simulink model "LMS0"  (R2018a)
settings: Solver=FixedStepDiscrete  StartTime=0.0  StopTime=3  RelTol=1e-3  EnableMultiTasking=on
libraries: dspvision x4
settings Model: Creator=gianc  LastModifiedBy=gianc
settings DataIOCC: LimitDataPoints=on  SaveOutput=off  SignalLogging=off  SaveTime=off
settings OptimizationCC: LifeSpan=inf
settings DebuggingCC: AlgebraicLoopMsg=error  SingleTaskRateTransMsg=error  AllowSymbolicDim=off  SFUnexpectedBacktrackingDiag=warning  SFNoUnconditionalDefaultTransitionDiag=warning  SFExecutionAtInitializationDiag=none
settings CodeAppCC: StateflowObjectComments=on
settings GRTTargetCC: TargetLangStandard=C89/C90 (ANSI)  GeneratePreprocessorConditionals=Disable all
settings ConfigComp: CovMetricSettings=dw  CovHtmlReporting=on  CovSaveCumulativeToWorkspaceVar=on  CovSaveSingleToWorkspaceVar=on  CovExternalEMLEnable=off  CovSFcnEnable=off

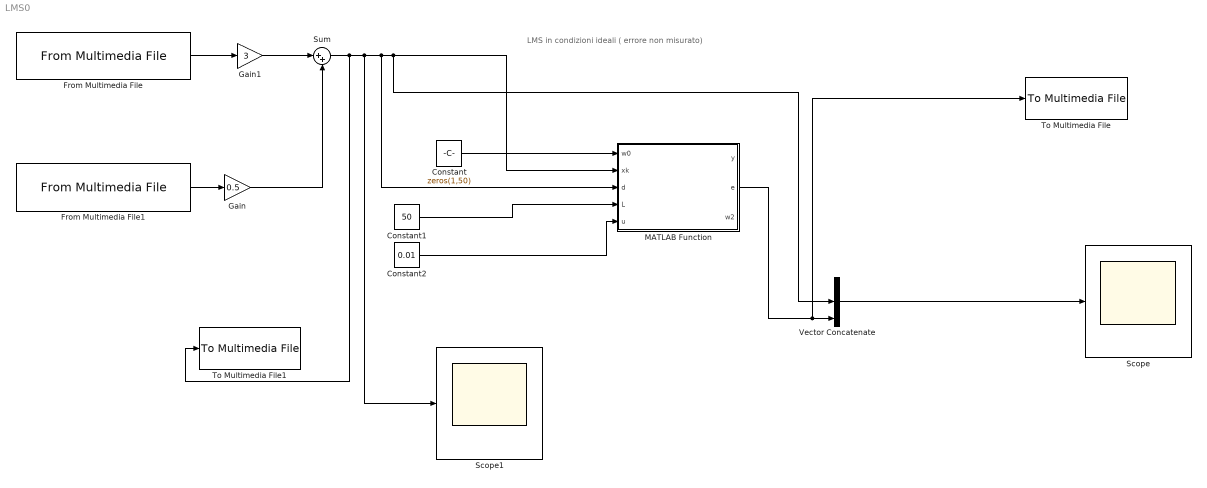
== system LMS0 ==
  note: LMS in condizioni ideali ( errore non misurato)
  Constant : Constant  Value=zeros(1,50)  VectorParams1D=off
  Constant1 : Constant  Value=50
  Constant2 : Constant  Value=0.01
  From Multimedia File : dspvision/From Multimedia File  inputFilename=C:\Users\gianc\Downloads\gun-gunshot-01.mp3  loop=on  numPlays=10  outputStreams=Audio only  videoDataType=single  audioDataType=double  inheritSampleTime=off  userDefinedSampleTime=1/22050  noAudioOutput=off  isIntensityVideo=off  fourcc=RGB  colorVideoFormat=Separate color signals  outputEOF=off  dataOrg=Column-major  audioFrameSize=1  computeAudioFrameSize=off  outSamplingMode=Sample based
      settings: SourceProductBaseCode=VP
  From Multimedia File1 : dspvision/From Multimedia File  inputFilename=speech_dft.mp3  loop=on  numPlays=10  outputStreams=Audio only  videoDataType=single  audioDataType=double  inheritSampleTime=on  userDefinedSampleTime=1/30  noAudioOutput=off  isIntensityVideo=off  fourcc=RGB  colorVideoFormat=Separate color signals  outputEOF=off  dataOrg=Column-major  audioFrameSize=1  computeAudioFrameSize=off  outSamplingMode=Sample based
      settings: SourceProductBaseCode=VP
  Gain : Gain  Gain=0.5
  Gain1 : Gain  Gain=3
  MATLAB Function : MATLAB Function  TreatAsAtomicUnit=on
  Scope : Scope
  Scope1 : Scope
  Sum : Sum  Inputs=|++
  To Multimedia File : dspvision/To Multimedia File  outputFilename=C:\Users\gianc\Desktop\output.wav  streamSelection=Audio only  videoCompressor=None (uncompressed)  audioCompressor=None (uncompressed)  imagePorts=Separate color signals  fileType=WAV  audioDatatype=16-bit integer  fourcc=RGB  videoQuality=75  mj2000CompFactor=10
      settings: SourceProductName=Computer Vision System Toolbox  SourceProductBaseCode=VP
  To Multimedia File1 : dspvision/To Multimedia File  outputFilename=C:\Users\gianc\Desktop\outputx.wav  streamSelection=Audio only  videoCompressor=None (uncompressed)  audioCompressor=None (uncompressed)  imagePorts=Separate color signals  fileType=WAV  audioDatatype=16-bit integer  fourcc=RGB  videoQuality=75  mj2000CompFactor=10
      settings: SourceProductName=Computer Vision System Toolbox  SourceProductBaseCode=VP
  Vector Concatenate : Concatenate  NumInputs=3
  wires:
  Constant/1 -> MATLAB Function/1(w0)
  Constant1/1 -> MATLAB Function/4(L)
  Constant2/1 -> MATLAB Function/5(u)
  Sum/1 -> To Multimedia File1/1, Scope1/1, MATLAB Function/3(d), Vector Concatenate/2, MATLAB Function/2(xk)
  From Multimedia File1/1 -> Gain/1
  Gain/1 -> Sum/2
  From Multimedia File/1 -> Gain1/1
  Gain1/1 -> Sum/1
  Vector Concatenate/1 -> Scope/1
  MATLAB Function/2(e) -> To Multimedia File/1, Vector Concatenate/3

== matlab function LMS0/MATLAB Function ==
  data: w0 input; y output; xk input; d input; L input; u input; e output; w2 output
%y=output filter (anti noise)
%w=weights vector 1xL
%x=input vector 1xL
%xk=sampled input at time k
%d=wanted signal (ideal is x but we have d=P*x)

function [y,e,w2] = LMS(w0,xk,d,L,u)

%global variables
[sizeD,~]=size(d);
y=zeros(sizeD,1);
%yneg=zeros(sizeD,1);
e=zeros(sizeD,1);
persistent cnt
persistent x
persistent w

for i=1:sizeD
    
if isempty(cnt)
    cnt=1;
else
    cnt=cnt+1;
end

if isempty(x)
    x=zeros(1,L);
end

if isempty(w)
    w=w0;
end

x=[xk(i,1) x(1:(L-1))]; %shift and add xk (FIFO)
y(i)= w*(x');
e(i) = d(i,1)-y(i); % e measured with a sensor or estimated
w = w + u*x*e(i); %refresh w for the next iteration

%yneg(i)=0-y(i);
end
w2=w;

end
